simulink model "DualSixPhaseInverter"  (R2018b)
settings: Solver=ode23tb  StartTime=0.0  StopTime=0.06  MaxStep=1e-6  RelTol=1e-4
InitFcn:
  | Vm = 100;
  | f = 100;
  | Vdc1 = 200;
  | Vdc2 = 200;
  | ratio = Vdc1 / Vdc2;
  | tpwm = 1e-4;
  | Td = 2e-6;
  | R = 10;
  | L = 20e-3;
  | Vf = 1;
  | Vfd = 1;
libraries: powerlib x33, powerlib_meascontrol x24, simulink_extras x2, simulink x2
settings Model: Creator=chenhao  LastModifiedBy=chenhao

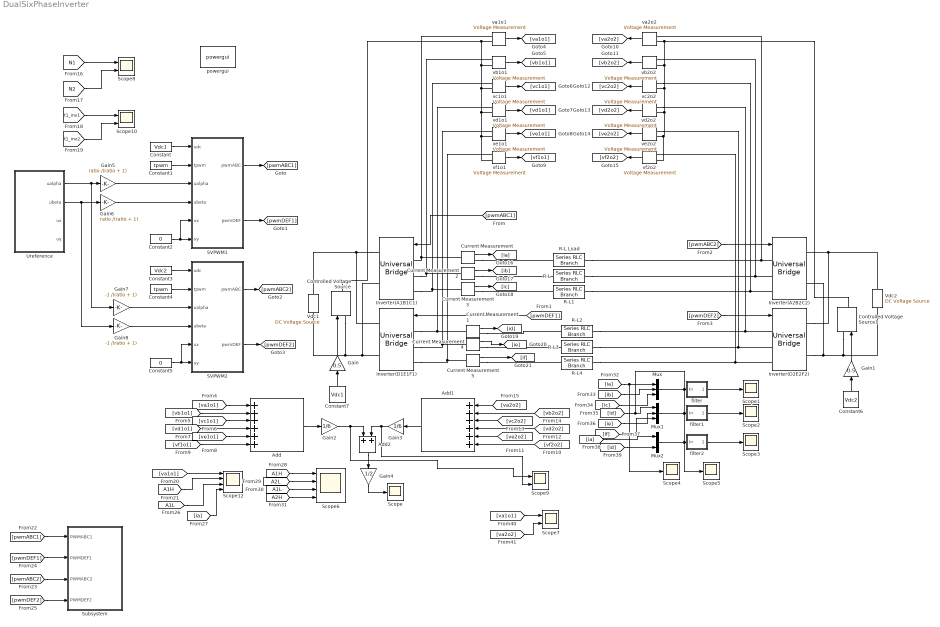
== system DualSixPhaseInverter ==
  Add : Sum  Inputs=++++++
  Add1 : Sum  Inputs=++++++
  Add2 : Sum
  Constant : Constant  Value=Vdc1
  Constant1 : Constant  Value=tpwm
  Constant2 : Constant  Value=0
  Constant3 : Constant  Value=Vdc2
  Constant4 : Constant  Value=tpwm
  Constant5 : Constant  Value=0
  Constant6 : Constant  Value=Vdc2
  Constant7 : Constant  Value=Vdc1
  Controlled Voltage Source : powerlib/Electrical Sources/Controlled Voltage Source  Initialize=on  Source_Type=AC  Amplitude=0  Phase=0  Frequency=0  Measurements=None
  Controlled Voltage Source1 : powerlib/Electrical Sources/Controlled Voltage Source  Initialize=on  Source_Type=AC  Amplitude=0  Phase=0  Frequency=0  Measurements=None
  Current Measurement{,1..5} (6 alike) : powerlib/Measurements/Current Measurement  PhasorSimulation=off  OutputType=Complex  PSBequivalent=0
  Gain : Gain  Gain=0.5
  Gain1 : Gain  Gain=0.5
  Gain2 : Gain  Gain=1/6
  Gain3 : Gain  Gain=1/6
  Gain4 : Gain  Gain=1/2
  Gain5 : Gain  Gain=ratio /(ratio + 1)
  Gain6 : Gain  Gain=ratio /(ratio + 1)
  Gain7 : Gain  Gain=-1 /(ratio + 1)
  Gain8 : Gain  Gain=-1 /(ratio + 1)
  Inverter(A1B1C1) : powerlib/Power Electronics/Universal Bridge  Arms=3  SnubberResistance=1e5  SnubberCapacitance=inf  Device=IGBT / Diodes  Ron=1e-3  Lon=0  ForwardVoltages="[  Vf  Vfd  ]"  ForwardVoltage=0  GTOparameters=[ 10e-6 , 20e-6 ]  IGBTparameters=[ 1e-6 , 2e-6 ]  Measurements=None  Measurements_2=None  converterType=Rectifier
      settings: SourceProductName=Simscape Electrical
  Inverter(A2B2C2) : powerlib/Power Electronics/Universal Bridge  Arms=3  SnubberResistance=1e5  SnubberCapacitance=inf  Device=IGBT / Diodes  Ron=1e-3  Lon=0  ForwardVoltages="[  Vf  Vfd  ]"  ForwardVoltage=0  GTOparameters=[ 10e-6 , 20e-6 ]  IGBTparameters=[ 1e-6 , 2e-6 ]  Measurements=None  Measurements_2=None  converterType=Rectifier
      settings: SourceProductName=Simscape Electrical
  Inverter(D1E1F1) : powerlib/Power Electronics/Universal Bridge  Arms=3  SnubberResistance=1e5  SnubberCapacitance=inf  Device=IGBT / Diodes  Ron=1e-3  Lon=0  ForwardVoltages="[  Vf  Vfd  ]"  ForwardVoltage=0  GTOparameters=[ 10e-6 , 20e-6 ]  IGBTparameters=[ 1e-6 , 2e-6 ]  Measurements=None  Measurements_2=None  converterType=Rectifier
      settings: SourceProductName=Simscape Electrical
  Inverter(D2E2F2) : powerlib/Power Electronics/Universal Bridge  Arms=3  SnubberResistance=1e5  SnubberCapacitance=inf  Device=IGBT / Diodes  Ron=1e-3  Lon=0  ForwardVoltages="[  Vf  Vfd  ]"  ForwardVoltage=0  GTOparameters=[ 10e-6 , 20e-6 ]  IGBTparameters=[ 1e-6 , 2e-6 ]  Measurements=None  Measurements_2=None  converterType=Rectifier
      settings: SourceProductName=Simscape Electrical
  Mux : Mux  Inputs=3
  Mux1 : Mux  Inputs=3
  Mux2 : Mux  Inputs=2
  R-L{,1..4} (5 alike) : powerlib/Elements/Series RLC Branch  LConnTagsString=__new0  RConnTagsString=__new0  BranchType=RL  Resistance=R  Inductance=L  SetiL0=off  InitialCurrent=0  Capacitance=[]  Setx0=off  InitialVoltage=0  Measurements=None
      settings: SourceProductName=Simscape Electrical
  R-L Load : powerlib/Elements/Series RLC Branch  LConnTagsString=__new0  RConnTagsString=__new0  BranchType=RL  Resistance=R  Inductance=L  SetiL0=off  InitialCurrent=0  Capacitance=[]  Setx0=off  InitialVoltage=0  Measurements=None
      settings: SourceProductName=Simscape Electrical
  SVPWM1 : Subsystem
  SVPWM2 : Subsystem
  Scope{,1..5} (6 alike) : Scope
  Scope{7..10} (4 alike) : Scope  NumInputPorts=2
  Scope12 : Scope  NumInputPorts=4
  Scope6 : Scope  NumInputPorts=4
  Subsystem : Subsystem
  Ureference : Subsystem
  Vdc1 : powerlib/Electrical Sources/DC Voltage Source  Amplitude=Vdc1  Measurements=None
      settings: SourceProductName=Simscape Electrical
  Vdc2 : powerlib/Electrical Sources/DC Voltage Source  Amplitude=Vdc2  Measurements=None
      settings: SourceProductName=Simscape Electrical
  filter : Subsystem
  filter1 : Subsystem
  filter2 : Subsystem
  powergui : powerlib/powergui  Priority=1  SimulationMode=Continuous  SampleTime=50e-6  frequency=60  Iterations=50  frequencyindice=0  Pbase=100e6  ErrMax=1e-4  UnitsV=kV  UnitsW=MW  buscounter=0  FunctionMessages=off  echomessages=off  EnableUseOfTLC=off  CurrentSourceSwitches=on  DisableSnubberDevices=off  DisableRonSwitches=off  DisableVfSwitches=off  DisplayEquations=off  SolverType=Tustin/Backward Euler (TBE)  Interpol=off  ExternalGateDelay=off  methode=off  Ts=100  x0status=blocks  SPID=off  SwTol=0  HookPort=off  RestoreLinks=warning  ResistiveCurrentMeasurement=off  Frange=[0:2:500]  Ylog=off  Xlog=on  ShowGrid=off  save=off  variable=ZData  structure=iA  ZoomFFT=off  StartTime=0.02  cycles=2  DisplayStyle=1  fundamental=100  FreqAxis=off  MaxFrequency=2000  frequencyindicesteady=1  RmsSteady=1  display=off
  va1o1 : powerlib/Measurements/Voltage Measurement  PhasorSimulation=off  OutputType=Complex  PSBequivalent=0
  va2o2 : powerlib/Measurements/Voltage Measurement  PhasorSimulation=off  OutputType=Complex  PSBequivalent=0
  vb1o1 : powerlib/Measurements/Voltage Measurement  PhasorSimulation=off  OutputType=Complex  PSBequivalent=0
  vb2o2 : powerlib/Measurements/Voltage Measurement  PhasorSimulation=off  OutputType=Complex  PSBequivalent=0
  vc1o1 : powerlib/Measurements/Voltage Measurement  PhasorSimulation=off  OutputType=Complex  PSBequivalent=0
  vc2o2 : powerlib/Measurements/Voltage Measurement  PhasorSimulation=off  OutputType=Complex  PSBequivalent=0
  vd1o1 : powerlib/Measurements/Voltage Measurement  PhasorSimulation=off  OutputType=Complex  PSBequivalent=0
  vd2o2 : powerlib/Measurements/Voltage Measurement  PhasorSimulation=off  OutputType=Complex  PSBequivalent=0
  ve1o1 : powerlib/Measurements/Voltage Measurement  PhasorSimulation=off  OutputType=Complex  PSBequivalent=0
  ve2o2 : powerlib/Measurements/Voltage Measurement  PhasorSimulation=off  OutputType=Complex  PSBequivalent=0
  vf1o1 : powerlib/Measurements/Voltage Measurement  PhasorSimulation=off  OutputType=Complex  PSBequivalent=0
  vf2o2 : powerlib/Measurements/Voltage Measurement  PhasorSimulation=off  OutputType=Complex  PSBequivalent=0
  wires:
  Constant/1 -> SVPWM1/1(udc)
  Constant1/1 -> SVPWM1/2(tpwm)
  Constant2/1 -> SVPWM1/6(uy), SVPWM1/5(ux)
  [pwmDEF1] -> Inverter(D1E1F1)/1
  [pwmABC1] -> Inverter(A1B1C1)/1
  Constant3/1 -> SVPWM2/1(udc)
  Constant4/1 -> SVPWM2/2(tpwm)
  Constant5/1 -> SVPWM2/5(ux), SVPWM2/6(uy)
  SVPWM2/1(pwmABC) -> [pwmABC2]
  Gain/1 -> Controlled Voltage Source/1
  Gain1/1 -> Controlled Voltage Source1/1
  va1o1/1 -> [va1o1]
  vb1o1/1 -> [vb1o1]
  vc1o1/1 -> [vc1o1]
  vd1o1/1 -> [vd1o1]
  ve1o1/1 -> [ve1o1]
  vf1o1/1 -> [vf1o1]
  vf2o2/1 -> [vf2o2]
  ve2o2/1 -> [ve2o2]
  vd2o2/1 -> [vd2o2]
  vc2o2/1 -> [vc2o2]
  vb2o2/1 -> [vb2o2]
  va2o2/1 -> [va2o2]
  [va1o1] -> Add/1
  [vb1o1] -> Add/2
  [vc1o1] -> Add/3
  [vd1o1] -> Add/4
  [ve1o1] -> Add/5
  [vf1o1] -> Add/6
  Add/1 -> Gain2/1
  Add1/1 -> Gain3/1
  [va2o2] -> Add1/1
  [vb2o2] -> Add1/2
  [vc2o2] -> Add1/3
  [vd2o2] -> Add1/4
  [ve2o2] -> Add1/5
  [vf2o2] -> Add1/6
  Add2/1 -> Gain4/1
  Gain4/1 -> Scope/1
  Ureference/1(ualpha) -> Gain7/1, Gain5/1
  Gain5/1 -> SVPWM1/3(ualpha)
  Ureference/2(ubeta) -> Gain8/1, Gain6/1
  Gain6/1 -> SVPWM1/4(ubeta)
  Mux/1 -> filter/1(In)
  filter/1(Out) -> Scope1/1
  Mux1/1 -> filter1/1(In)
  filter1/1(Out) -> Scope2/1
  Mux2/1 -> filter2/1(In)
  filter2/1(Out) -> Scope3/1
  [pwmABC2] -> Inverter(A2B2C2)/1
  [pwmDEF2] -> Inverter(D2E2F2)/1
  Gain8/1 -> SVPWM2/4(ubeta)
  Gain7/1 -> SVPWM2/3(ualpha)
  SVPWM1/1(pwmABC) -> [pwmABC1]
  [N1] -> Scope8/1
  [N2] -> Scope8/2
  SVPWM2/2(pwmDEF) -> [pwmDEF2]
  SVPWM1/2(pwmDEF) -> [pwmDEF1]
  Gain3/1 -> Scope9/2, Add2/2
  Gain2/1 -> Scope9/1, Add2/1
  Constant6/1 -> Gain1/1
  Constant7/1 -> Gain/1
  [t1_inv1] -> Scope10/1
  [t1_inv2] -> Scope10/2
  [va1o1] -> Scope12/1
  [A1H] -> Scope12/2
  [pwmABC1] -> Subsystem/1(PWMABC1)
  [pwmABC2] -> Subsystem/3(PWMABC2)
  [pwmDEF1] -> Subsystem/2(PWMDEF1)
  [pwmDEF2] -> Subsystem/4(PWMDEF2)
  [A1L] -> Scope12/3
  Current Measurement/1 -> [ia]
  Current Measurement2/1 -> [ib]
  Current Measurement3/1 -> [ic]
  Current Measurement1/1 -> [id]
  Current Measurement4/1 -> [ie]
  Current Measurement5/1 -> [if]
  [ia] -> Scope12/4
  [A1H] -> Scope6/1
  [A2L] -> Scope6/2
  [A1L] -> Scope6/3
  [A2H] -> Scope6/4
  [ia] -> Scope4/1, Mux/1
  [ib] -> Mux/2
  [ic] -> Mux/3
  [id] -> Scope5/1, Mux1/1
  [ie] -> Mux1/2
  [if] -> Mux1/3
  [ia] -> Mux2/1
  [id] -> Mux2/2
  [va1o1] -> Scope7/1
  [va2o2] -> Scope7/2
  connections:
  Inverter(A1B1C1)/RConn2 -- Vdc1/LConn1 -- Controlled Voltage Source/LConn1 -- Inverter(D1E1F1)/RConn2
  Inverter(D1E1F1)/LConn1 -- vd1o1/LConn1 -- Current Measurement1/LConn1
  Inverter(A1B1C1)/LConn1 -- Current Measurement/LConn1 -- va1o1/LConn1
  Inverter(A1B1C1)/RConn1 -- Vdc1/RConn1 -- Inverter(D1E1F1)/RConn1
  Inverter(D1E1F1)/LConn2 -- Current Measurement4/LConn1 -- ve1o1/LConn1
  Inverter(D1E1F1)/LConn3 -- Current Measurement5/LConn1 -- vf1o1/LConn1
  Inverter(A1B1C1)/LConn3 -- Current Measurement3/LConn1 -- vc1o1/LConn1
  Inverter(A1B1C1)/LConn2 -- Current Measurement2/LConn1 -- vb1o1/LConn1
  Inverter(D2E2F2)/RConn2 -- Vdc2/LConn1 -- Controlled Voltage Source1/LConn1 -- Inverter(A2B2C2)/RConn2
  Inverter(D2E2F2)/RConn1 -- Vdc2/RConn1 -- Inverter(A2B2C2)/RConn1
  vc2o2/LConn1 -- Inverter(A2B2C2)/LConn3 -- R-L1/RConn1
  Inverter(A2B2C2)/LConn2 -- R-L/RConn1 -- vb2o2/LConn1
  Inverter(A2B2C2)/LConn1 -- R-L Load/RConn1 -- va2o2/LConn1
  vd2o2/LConn1 -- Inverter(D2E2F2)/LConn1 -- R-L2/RConn1
  ve2o2/LConn1 -- Inverter(D2E2F2)/LConn2 -- R-L3/RConn1
  vf2o2/LConn1 -- R-L4/RConn1 -- Inverter(D2E2F2)/LConn3
  va1o1/LConn2 -- vf1o1/LConn2 -- ve1o1/LConn2 -- vd1o1/LConn2 -- vc1o1/LConn2 -- vb1o1/LConn2 -- Controlled Voltage Source/RConn1
  va2o2/LConn2 -- vf2o2/LConn2 -- ve2o2/LConn2 -- vd2o2/LConn2 -- vc2o2/LConn2 -- vb2o2/LConn2 -- Controlled Voltage Source1/RConn1
  Current Measurement/RConn1 -- R-L Load/LConn1
  Current Measurement1/RConn1 -- R-L2/LConn1
  Current Measurement2/RConn1 -- R-L/LConn1
  Current Measurement3/RConn1 -- R-L1/LConn1
  Current Measurement4/RConn1 -- R-L3/LConn1
  Current Measurement5/RConn1 -- R-L4/LConn1

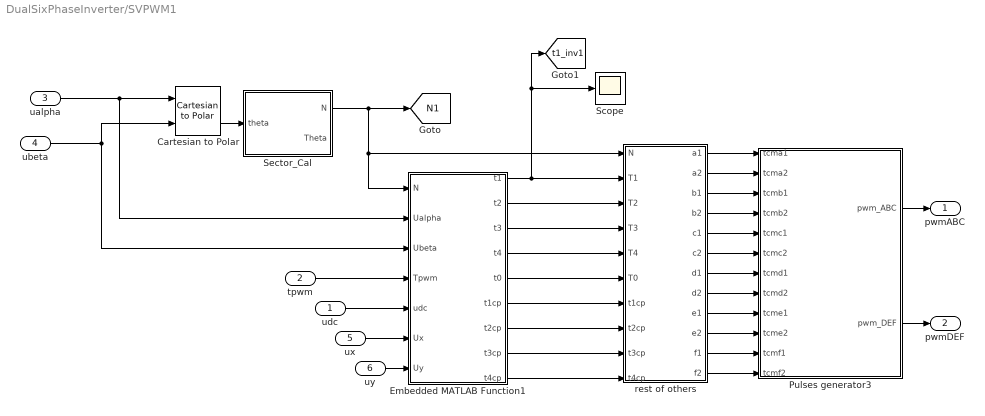
== system DualSixPhaseInverter/SVPWM1 ==
  udc : Inport
  tpwm : Inport  Port=2
  ualpha : Inport  Port=3
  ubeta : Inport  Port=4
  ux : Inport  Port=5
  uy : Inport  Port=6
  Cartesian to Polar : simulink_extras/Transformations/Cartesian to Polar
      settings: SourceProductName=Simulink
  Embedded MATLAB Function1 : MATLAB Function  TreatAsAtomicUnit=on
  Pulses generator3 : Subsystem
  Scope : Scope
  Sector_Cal : Subsystem
  rest of others : MATLAB Function  TreatAsAtomicUnit=on
  pwmABC : Outport
  pwmDEF : Outport  Port=2
  tag scope: N1=global, t1_inv1=global
  wires:
  tpwm/1 -> Embedded MATLAB Function1/4(Tpwm)
  ubeta/1 -> Cartesian to Polar/2, Embedded MATLAB Function1/3(Ubeta)
  ualpha/1 -> Cartesian to Polar/1, Embedded MATLAB Function1/2(Ualpha)
  ux/1 -> Embedded MATLAB Function1/6(Ux)
  uy/1 -> Embedded MATLAB Function1/7(Uy)
  udc/1 -> Embedded MATLAB Function1/5(udc)
  rest of others/12(f2) -> Pulses generator3/12(tcmf2)
  rest of others/11(f1) -> Pulses generator3/11(tcmf1)
  rest of others/9(e1) -> Pulses generator3/9(tcme1)
  rest of others/8(d2) -> Pulses generator3/8(tcmd2)
  rest of others/10(e2) -> Pulses generator3/10(tcme2)
  rest of others/2(a2) -> Pulses generator3/2(tcma2)
  rest of others/6(c2) -> Pulses generator3/6(tcmc2)
  rest of others/4(b2) -> Pulses generator3/4(tcmb2)
  rest of others/5(c1) -> Pulses generator3/5(tcmc1)
  rest of others/7(d1) -> Pulses generator3/7(tcmd1)
  rest of others/3(b1) -> Pulses generator3/3(tcmb1)
  rest of others/1(a1) -> Pulses generator3/1(tcma1)
  Embedded MATLAB Function1/1(t1) -> [t1_inv1], Scope/1, rest of others/2(T1)
  Embedded MATLAB Function1/2(t2) -> rest of others/3(T2)
  Embedded MATLAB Function1/3(t3) -> rest of others/4(T3)
  Embedded MATLAB Function1/4(t4) -> rest of others/5(T4)
  Embedded MATLAB Function1/5(t0) -> rest of others/6(T0)
  Embedded MATLAB Function1/6(t1cp) -> rest of others/7(t1cp)
  Embedded MATLAB Function1/7(t2cp) -> rest of others/8(t2cp)
  Embedded MATLAB Function1/8(t3cp) -> rest of others/9(t3cp)
  Embedded MATLAB Function1/9(t4cp) -> rest of others/10(t4cp)
  Cartesian to Polar/2 -> Sector_Cal/1(theta)
  Sector_Cal/1(N) -> [N1], rest of others/1(N), Embedded MATLAB Function1/1(N)
  Pulses generator3/1(pwm_ABC) -> pwmABC/1
  Pulses generator3/2(pwm_DEF) -> pwmDEF/1

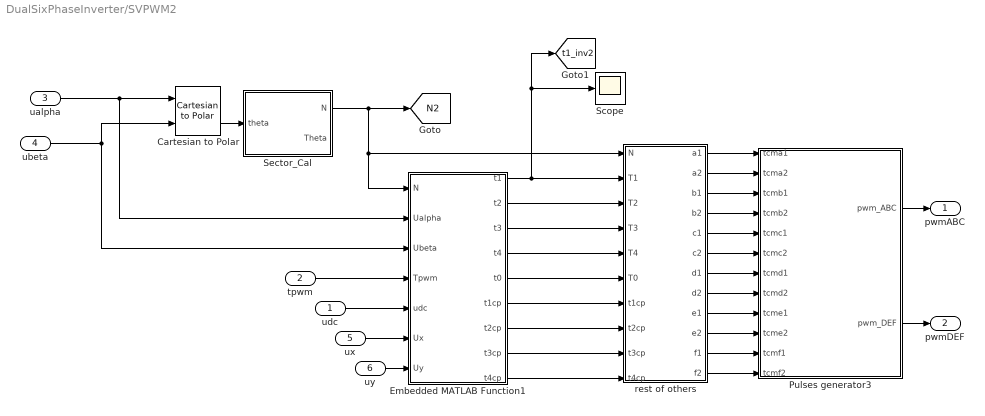
== system DualSixPhaseInverter/SVPWM2 ==
  udc : Inport
  tpwm : Inport  Port=2
  ualpha : Inport  Port=3
  ubeta : Inport  Port=4
  ux : Inport  Port=5
  uy : Inport  Port=6
  Cartesian to Polar : simulink_extras/Transformations/Cartesian to Polar
      settings: SourceProductName=Simulink
  Embedded MATLAB Function1 : MATLAB Function  TreatAsAtomicUnit=on
  Pulses generator3 : Subsystem
  Scope : Scope
  Sector_Cal : Subsystem
  rest of others : MATLAB Function  TreatAsAtomicUnit=on
  pwmABC : Outport
  pwmDEF : Outport  Port=2
  tag scope: N2=global, t1_inv2=global
  wires:
  Pulses generator3/2(pwm_DEF) -> pwmDEF/1
  Pulses generator3/1(pwm_ABC) -> pwmABC/1
  Sector_Cal/1(N) -> [N2], Embedded MATLAB Function1/1(N), rest of others/1(N)
  Cartesian to Polar/2 -> Sector_Cal/1(theta)
  Embedded MATLAB Function1/9(t4cp) -> rest of others/10(t4cp)
  Embedded MATLAB Function1/8(t3cp) -> rest of others/9(t3cp)
  Embedded MATLAB Function1/7(t2cp) -> rest of others/8(t2cp)
  Embedded MATLAB Function1/6(t1cp) -> rest of others/7(t1cp)
  Embedded MATLAB Function1/5(t0) -> rest of others/6(T0)
  Embedded MATLAB Function1/4(t4) -> rest of others/5(T4)
  Embedded MATLAB Function1/3(t3) -> rest of others/4(T3)
  Embedded MATLAB Function1/2(t2) -> rest of others/3(T2)
  Embedded MATLAB Function1/1(t1) -> rest of others/2(T1), [t1_inv2], Scope/1
  rest of others/1(a1) -> Pulses generator3/1(tcma1)
  rest of others/3(b1) -> Pulses generator3/3(tcmb1)
  rest of others/7(d1) -> Pulses generator3/7(tcmd1)
  rest of others/5(c1) -> Pulses generator3/5(tcmc1)
  rest of others/4(b2) -> Pulses generator3/4(tcmb2)
  rest of others/6(c2) -> Pulses generator3/6(tcmc2)
  rest of others/2(a2) -> Pulses generator3/2(tcma2)
  rest of others/10(e2) -> Pulses generator3/10(tcme2)
  rest of others/8(d2) -> Pulses generator3/8(tcmd2)
  rest of others/9(e1) -> Pulses generator3/9(tcme1)
  rest of others/11(f1) -> Pulses generator3/11(tcmf1)
  rest of others/12(f2) -> Pulses generator3/12(tcmf2)
  udc/1 -> Embedded MATLAB Function1/5(udc)
  uy/1 -> Embedded MATLAB Function1/7(Uy)
  ux/1 -> Embedded MATLAB Function1/6(Ux)
  ualpha/1 -> Embedded MATLAB Function1/2(Ualpha), Cartesian to Polar/1
  ubeta/1 -> Embedded MATLAB Function1/3(Ubeta), Cartesian to Polar/2
  tpwm/1 -> Embedded MATLAB Function1/4(Tpwm)

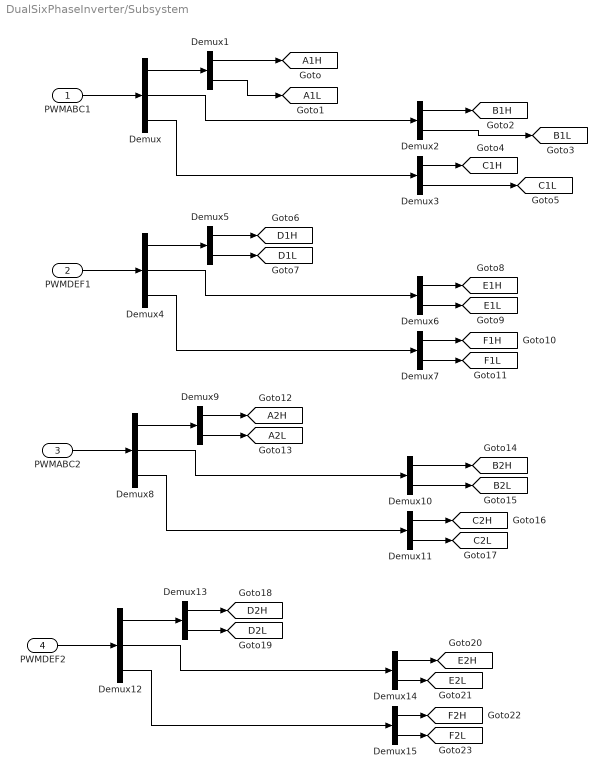
== system DualSixPhaseInverter/Subsystem ==
  PWMABC1 : Inport
  PWMDEF1 : Inport  Port=2
  PWMABC2 : Inport  Port=3
  PWMDEF2 : Inport  Port=4
  Demux{,4,8,12} (4 alike) : Demux  Outputs=3
  Demux{1..3,5..7,9..11,13..15} (12 alike) : Demux  Outputs=2
  tag scope: A1H=global, A1L=global, A2H=global, A2L=global, B1H=global, B1L=global, B2H=global, B2L=global, C1H=global, C1L=global, C2H=global, C2L=global, D1H=global, D1L=global, D2H=global, D2L=global, E1H=global, E1L=global, E2H=global, E2L=global, F1H=global, F1L=global, F2H=global, F2L=global
  wires:
  PWMABC1/1 -> Demux/1
  Demux/1 -> Demux1/1
  Demux/2 -> Demux2/1
  Demux/3 -> Demux3/1
  Demux4/3 -> Demux7/1
  Demux4/2 -> Demux6/1
  Demux4/1 -> Demux5/1
  PWMDEF1/1 -> Demux4/1
  PWMABC2/1 -> Demux8/1
  Demux8/1 -> Demux9/1
  Demux8/2 -> Demux10/1
  Demux8/3 -> Demux11/1
  Demux12/3 -> Demux15/1
  Demux12/2 -> Demux14/1
  Demux12/1 -> Demux13/1
  PWMDEF2/1 -> Demux12/1
  Demux1/1 -> [A1H]
  Demux1/2 -> [A1L]
  Demux2/1 -> [B1H]
  Demux2/2 -> [B1L]
  Demux3/1 -> [C1H]
  Demux3/2 -> [C1L]
  Demux5/1 -> [D1H]
  Demux5/2 -> [D1L]
  Demux6/1 -> [E1H]
  Demux6/2 -> [E1L]
  Demux7/1 -> [F1H]
  Demux7/2 -> [F1L]
  Demux9/1 -> [A2H]
  Demux9/2 -> [A2L]
  Demux10/1 -> [B2H]
  Demux10/2 -> [B2L]
  Demux11/1 -> [C2H]
  Demux11/2 -> [C2L]
  Demux13/1 -> [D2H]
  Demux13/2 -> [D2L]
  Demux14/1 -> [E2H]
  Demux14/2 -> [E2L]
  Demux15/1 -> [F2H]
  Demux15/2 -> [F2L]

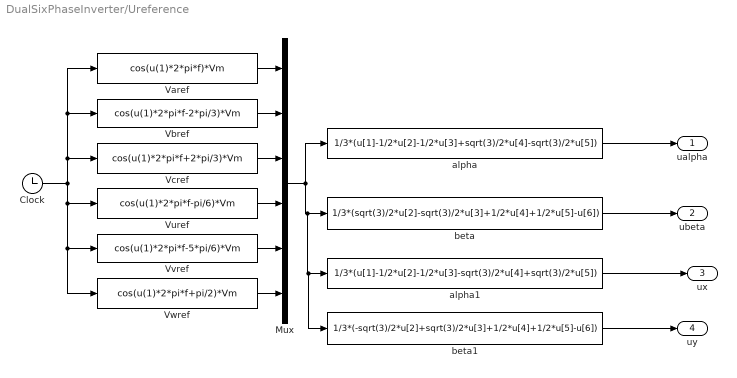
== system DualSixPhaseInverter/Ureference ==
  Clock : Clock
  Mux : Mux  Inputs=6
  Varef : Fcn  Expr=cos(u(1)*2*pi*f)*Vm
  Vbref : Fcn  Expr=cos(u(1)*2*pi*f-2*pi/3)*Vm
  Vcref : Fcn  Expr=cos(u(1)*2*pi*f+2*pi/3)*Vm
  Vuref : Fcn  Expr=cos(u(1)*2*pi*f-pi/6)*Vm
  Vvref : Fcn  Expr=cos(u(1)*2*pi*f-5*pi/6)*Vm
  Vwref : Fcn  Expr=cos(u(1)*2*pi*f+pi/2)*Vm
  alpha : Fcn  Expr=1/3*(u[1]-1/2*u[2]-1/2*u[3]+sqrt(3)/2*u[4]-sqrt(3)/2*u[5])
  alpha1 : Fcn  Expr=1/3*(u[1]-1/2*u[2]-1/2*u[3]-sqrt(3)/2*u[4]+sqrt(3)/2*u[5])
  beta : Fcn  Expr=1/3*(sqrt(3)/2*u[2]-sqrt(3)/2*u[3]+1/2*u[4]+1/2*u[5]-u[6])
  beta1 : Fcn  Expr=1/3*(-sqrt(3)/2*u[2]+sqrt(3)/2*u[3]+1/2*u[4]+1/2*u[5]-u[6])
  ualpha : Outport
  ubeta : Outport  Port=2
  ux : Outport  Port=3
  uy : Outport  Port=4
  wires:
  Vwref/1 -> Mux/6
  Vuref/1 -> Mux/4
  Vbref/1 -> Mux/2
  Vvref/1 -> Mux/5
  Varef/1 -> Mux/1
  Vcref/1 -> Mux/3
  Mux/1 -> alpha/1, beta1/1, alpha1/1, beta/1
  Clock/1 -> Varef/1, Vbref/1, Vcref/1, Vwref/1, Vvref/1, Vuref/1
  alpha/1 -> ualpha/1
  beta/1 -> ubeta/1
  alpha1/1 -> ux/1
  beta1/1 -> uy/1

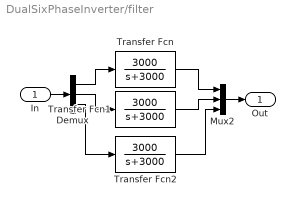
== system DualSixPhaseInverter/filter ==
  In : Inport
  Demux : Demux  Outputs=3
  Mux2 : Mux  Inputs=3
  Transfer Fcn : TransferFcn  Numerator=[3000]  Denominator=[1 3000]
  Transfer Fcn1 : TransferFcn  Numerator=[3000]  Denominator=[1 3000]
  Transfer Fcn2 : TransferFcn  Numerator=[3000]  Denominator=[1 3000]
  Out : Outport
  wires:
  Demux/1 -> Transfer Fcn/1
  Demux/2 -> Transfer Fcn1/1
  Transfer Fcn1/1 -> Mux2/2
  Transfer Fcn/1 -> Mux2/1
  In/1 -> Demux/1
  Mux2/1 -> Out/1
  Demux/3 -> Transfer Fcn2/1
  Transfer Fcn2/1 -> Mux2/3

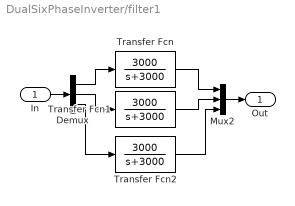
== system DualSixPhaseInverter/filter1 ==
  In : Inport
  Demux : Demux  Outputs=3
  Mux2 : Mux  Inputs=3
  Transfer Fcn : TransferFcn  Numerator=[3000]  Denominator=[1 3000]
  Transfer Fcn1 : TransferFcn  Numerator=[3000]  Denominator=[1 3000]
  Transfer Fcn2 : TransferFcn  Numerator=[3000]  Denominator=[1 3000]
  Out : Outport
  wires:
  Transfer Fcn2/1 -> Mux2/3
  Demux/3 -> Transfer Fcn2/1
  Mux2/1 -> Out/1
  In/1 -> Demux/1
  Transfer Fcn/1 -> Mux2/1
  Transfer Fcn1/1 -> Mux2/2
  Demux/2 -> Transfer Fcn1/1
  Demux/1 -> Transfer Fcn/1

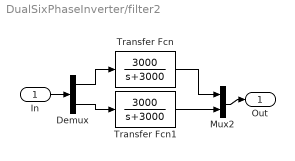
== system DualSixPhaseInverter/filter2 ==
  In : Inport
  Demux : Demux  Outputs=2
  Mux2 : Mux  Inputs=2
  Transfer Fcn : TransferFcn  Numerator=[3000]  Denominator=[1 3000]
  Transfer Fcn1 : TransferFcn  Numerator=[3000]  Denominator=[1 3000]
  Out : Outport
  wires:
  Demux/1 -> Transfer Fcn/1
  Demux/2 -> Transfer Fcn1/1
  Transfer Fcn1/1 -> Mux2/2
  Transfer Fcn/1 -> Mux2/1
  In/1 -> Demux/1
  Mux2/1 -> Out/1

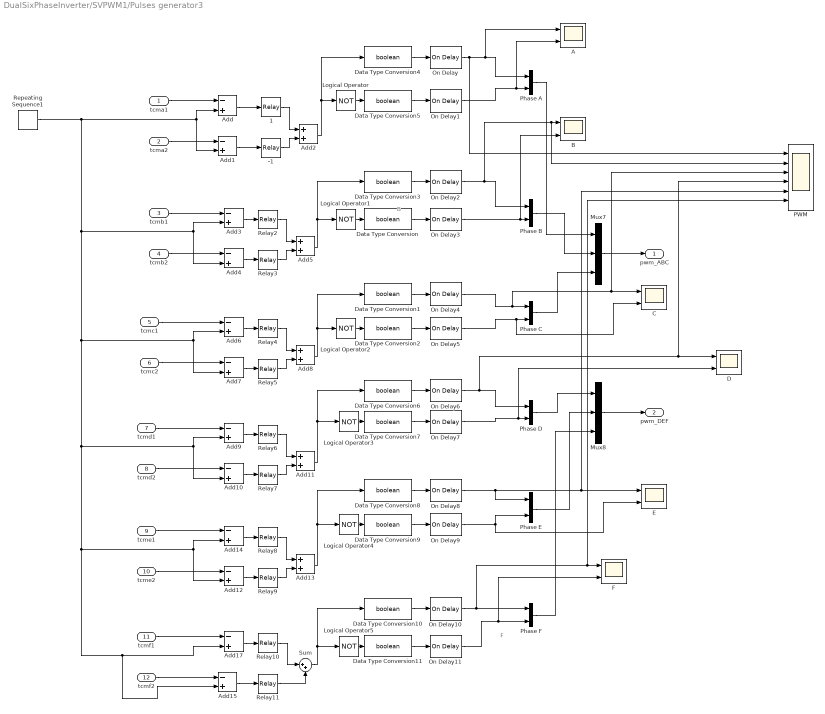
== system DualSixPhaseInverter/SVPWM1/Pulses generator3 ==
  note: B
  note: F
  tcma1 : Inport
  tcma2 : Inport  Port=2
  tcmb1 : Inport  Port=3
  tcmb2 : Inport  Port=4
  tcmc1 : Inport  Port=5
  tcmc2 : Inport  Port=6
  tcmd1 : Inport  Port=7
  tcmd2 : Inport  Port=8
  tcme1 : Inport  Port=9
  tcme2 : Inport  Port=10
  tcmf1 : Inport  Port=11
  tcmf2 : Inport  Port=12
  -1 : Relay  OnOutputValue=-1
  1 : Relay
  A : Scope  NumInputPorts=2
  Add{,1,3..4,6..7,9..10,12,14..15,17} (12 alike) : Sum  Inputs=-+
  Add{2,5,8,11,13} (5 alike) : Sum
  B : Scope  NumInputPorts=2
  C : Scope  NumInputPorts=2
  D : Scope  NumInputPorts=2
  Data Type Conversion{,1..11} (12 alike) : DataTypeConversion  OutDataTypeStr=boolean
  E : Scope  NumInputPorts=2
  F : Scope  NumInputPorts=2
  Logical Operator{,1..5} (6 alike) : Logic  Operator=NOT  AllPortsSameDT=off  OutDataTypeStr=boolean
  Mux7 : Mux  Inputs=3
  Mux8 : Mux  Inputs=3
  On Delay{,1..11} (12 alike) : powerlib_meascontrol/Logic/On Delay  DelayType=On delay  delay=Td  ic=0  Ts=0
      settings: SourceProductName=Simscape Power Systems
  PWM : Scope  NumInputPorts=6
  Phase A : Mux  Inputs=2
  Phase B : Mux  Inputs=2
  Phase C : Mux  Inputs=2
  Phase D : Mux  Inputs=2
  Phase E : Mux  Inputs=2
  Phase F : Mux  Inputs=2
  Relay{2,4,6,8,10} (5 alike) : Relay
  Relay{3,5,7,9,11} (5 alike) : Relay  OnOutputValue=-1
  Repeating Sequence1 : simulink/Sources/Repeating Sequence  rep_seq_t=[0 tpwm]  rep_seq_y=[0 tpwm]
  Sum : Sum  Inputs=|++
  pwm_ABC : Outport
  pwm_DEF : Outport  Port=2
  wires:
  On Delay11/1 -> F/2, Phase F/2
  Data Type Conversion11/1 -> On Delay11/1
  On Delay10/1 -> PWM/6, F/1, Phase F/1
  Data Type Conversion10/1 -> On Delay10/1
  On Delay9/1 -> E/2, Phase E/2
  Data Type Conversion9/1 -> On Delay9/1
  On Delay8/1 -> Phase E/1, PWM/5, E/1
  Data Type Conversion8/1 -> On Delay8/1
  On Delay7/1 -> D/2, Phase D/2
  Data Type Conversion7/1 -> On Delay7/1
  On Delay6/1 -> PWM/4, D/1, Phase D/1
  Data Type Conversion6/1 -> On Delay6/1
  On Delay5/1 -> C/2, Phase C/2
  Data Type Conversion2/1 -> On Delay5/1
  On Delay4/1 -> PWM/3, C/1, Phase C/1
  Data Type Conversion1/1 -> On Delay4/1
  On Delay2/1 -> PWM/2, B/1, Phase B/1
  On Delay3/1 -> B/2, Phase B/2
  Data Type Conversion/1 -> On Delay3/1
  Data Type Conversion3/1 -> On Delay2/1
  On Delay1/1 -> A/2, Phase A/2
  Data Type Conversion5/1 -> On Delay1/1
  On Delay/1 -> A/1, Phase A/1, PWM/1
  Data Type Conversion4/1 -> On Delay/1
  Logical Operator3/1 -> Data Type Conversion7/1
  Logical Operator2/1 -> Data Type Conversion2/1
  Logical Operator/1 -> Data Type Conversion5/1
  Logical Operator1/1 -> Data Type Conversion/1
  Logical Operator4/1 -> Data Type Conversion9/1
  Add5/1 -> Logical Operator1/1, Data Type Conversion3/1
  Add2/1 -> Logical Operator/1, Data Type Conversion4/1
  Mux8/1 -> pwm_DEF/1
  Mux7/1 -> pwm_ABC/1
  Sum/1 -> Data Type Conversion10/1, Logical Operator5/1
  Add13/1 -> Data Type Conversion8/1, Logical Operator4/1
  Add11/1 -> Data Type Conversion6/1, Logical Operator3/1
  Add8/1 -> Data Type Conversion1/1, Logical Operator2/1
  Logical Operator5/1 -> Data Type Conversion11/1
  tcmf2/1 -> Add15/1
  Relay11/1 -> Sum/2
  Relay10/1 -> Sum/1
  Add17/1 -> Relay10/1
  tcmf1/1 -> Add17/1
  tcme2/1 -> Add12/1
  Relay9/1 -> Add13/2
  Relay8/1 -> Add13/1
  Add12/1 -> Relay9/1
  Add14/1 -> Relay8/1
  tcme1/1 -> Add14/1
  tcmd2/1 -> Add10/1
  Relay7/1 -> Add11/2
  Relay6/1 -> Add11/1
  Add10/1 -> Relay7/1
  Add9/1 -> Relay6/1
  tcmd1/1 -> Add9/1
  tcmc2/1 -> Add7/1
  Relay5/1 -> Add8/2
  Relay4/1 -> Add8/1
  Add7/1 -> Relay5/1
  Add6/1 -> Relay4/1
  tcmb2/1 -> Add4/1
  Relay3/1 -> Add5/2
  Relay2/1 -> Add5/1
  Add4/1 -> Relay3/1
  Add3/1 -> Relay2/1
  tcma1/1 -> Add/1
  -1/1 -> Add2/2
  1/1 -> Add2/1
  Add1/1 -> -1/1
  Add/1 -> 1/1
  Repeating Sequence1/1 -> Add15/2, Add17/2, Add12/2, Add14/2, Add9/2, Add10/2, Add7/2, Add6/2, Add3/2, Add4/2, Add1/2, Add/2
  tcma2/1 -> Add1/1
  tcmb1/1 -> Add3/1
  tcmc1/1 -> Add6/1
  Add15/1 -> Relay11/1
  Phase A/1 -> Mux7/1
  Phase B/1 -> Mux7/2
  Phase C/1 -> Mux7/3
  Phase D/1 -> Mux8/1
  Phase E/1 -> Mux8/2
  Phase F/1 -> Mux8/3

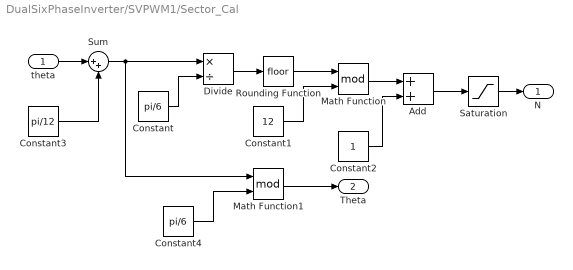
== system DualSixPhaseInverter/SVPWM1/Sector_Cal ==
  theta : Inport
  Add : Sum
  Constant : Constant  Value=pi/6
  Constant1 : Constant  Value=12
  Constant2 : Constant
  Constant3 : Constant  Value=pi/12
  Constant4 : Constant  Value=pi/6
  Divide : Product  Inputs=*/
  Math Function : Math  Operator=mod  SaturateOnIntegerOverflow=on
  Math Function1 : Math  Operator=mod  SaturateOnIntegerOverflow=on
  Rounding Function : Rounding
  Saturation : Saturate  UpperLimit=12  LowerLimit=1
  Sum : Sum  Inputs=|++
  N : Outport
  Theta : Outport  Port=2
  wires:
  Constant/1 -> Divide/2
  Divide/1 -> Rounding Function/1
  Rounding Function/1 -> Math Function/1
  Constant1/1 -> Math Function/2
  Math Function/1 -> Add/1
  Constant2/1 -> Add/2
  Add/1 -> Saturation/1
  Saturation/1 -> N/1
  theta/1 -> Sum/1
  Sum/1 -> Math Function1/1, Divide/1
  Constant3/1 -> Sum/2
  Constant4/1 -> Math Function1/2
  Math Function1/1 -> Theta/1

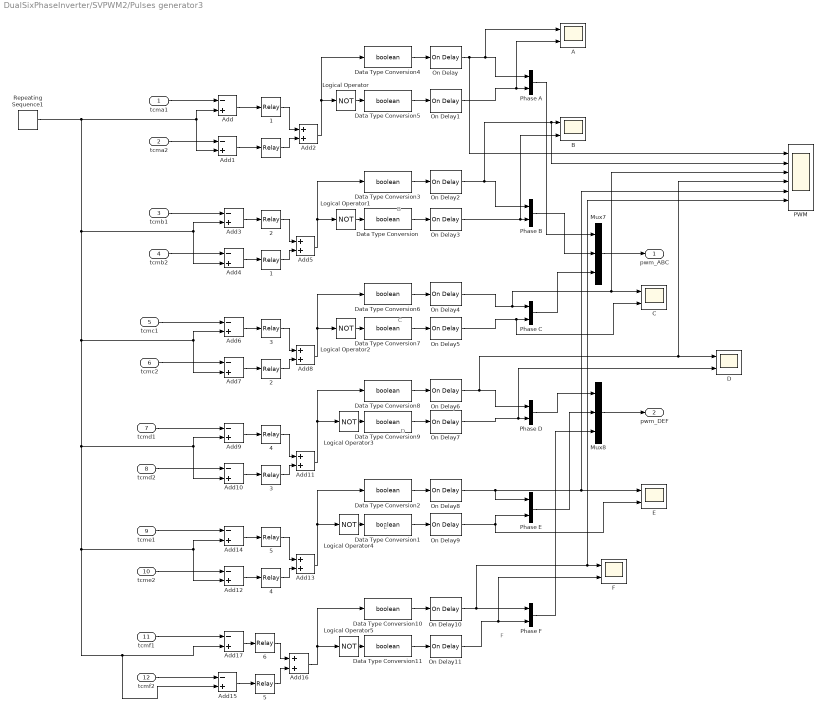
== system DualSixPhaseInverter/SVPWM2/Pulses generator3 ==
  note: F
  note: E
  note: D
  note: C
  note: B
  tcma1 : Inport
  tcma2 : Inport  Port=2
  tcmb1 : Inport  Port=3
  tcmb2 : Inport  Port=4
  tcmc1 : Inport  Port=5
  tcmc2 : Inport  Port=6
  tcmd1 : Inport  Port=7
  tcmd2 : Inport  Port=8
  tcme1 : Inport  Port=9
  tcme2 : Inport  Port=10
  tcmf1 : Inport  Port=11
  tcmf2 : Inport  Port=12
   {,1..5} (6 alike) : Relay
  {1..6} (6 alike) : Relay  OnOutputValue=0  OffOutputValue=1
  A : Scope  NumInputPorts=2
  Add{,1,3..4,6..7,9..10,12,14..15,17} (12 alike) : Sum  Inputs=-+
  Add{2,5,8,11,13,16} (6 alike) : Sum
  B : Scope  NumInputPorts=2
  C : Scope  NumInputPorts=2
  D : Scope  NumInputPorts=2
  Data Type Conversion{,1..11} (12 alike) : DataTypeConversion  OutDataTypeStr=boolean
  E : Scope  NumInputPorts=2
  F : Scope  NumInputPorts=2
  Logical Operator{,1..5} (6 alike) : Logic  Operator=NOT  AllPortsSameDT=off  OutDataTypeStr=boolean
  Mux7 : Mux  Inputs=3
  Mux8 : Mux  Inputs=3
  On Delay{,1..11} (12 alike) : powerlib_meascontrol/Logic/On Delay  DelayType=On delay  delay=Td  ic=0  Ts=0
      settings: SourceProductName=Simscape Power Systems
  PWM : Scope  NumInputPorts=6
  Phase A : Mux  Inputs=2
  Phase B : Mux  Inputs=2
  Phase C : Mux  Inputs=2
  Phase D : Mux  Inputs=2
  Phase E : Mux  Inputs=2
  Phase F : Mux  Inputs=2
  Repeating Sequence1 : simulink/Sources/Repeating Sequence  rep_seq_t=[0 tpwm]  rep_seq_y=[0 tpwm]
  pwm_ABC : Outport
  pwm_DEF : Outport  Port=2
  wires:
  Phase F/1 -> Mux8/3
  Phase E/1 -> Mux8/2
  Phase D/1 -> Mux8/1
  Phase C/1 -> Mux7/3
  Phase B/1 -> Mux7/2
  Phase A/1 -> Mux7/1
  tcmc1/1 -> Add6/1
  tcmb1/1 -> Add3/1
  tcma2/1 -> Add1/1
  Repeating Sequence1/1 -> Add/2, Add1/2, Add4/2, Add3/2, Add6/2, Add7/2, Add10/2, Add9/2, Add14/2, Add12/2, Add17/2, Add15/2
  Add/1 -> 1/1
  Add1/1 -> " "/1
  1/1 -> Add2/1
  " "/1 -> Add2/2
  tcma1/1 -> Add/1
  tcmb2/1 -> Add4/1
  tcmc2/1 -> Add7/1
  tcmd1/1 -> Add9/1
  tcmd2/1 -> Add10/1
  tcme1/1 -> Add14/1
  tcme2/1 -> Add12/1
  tcmf1/1 -> Add17/1
  tcmf2/1 -> Add15/1
  Logical Operator5/1 -> Data Type Conversion11/1
  Add8/1 -> Data Type Conversion6/1, Logical Operator2/1
  Add11/1 -> Data Type Conversion8/1, Logical Operator3/1
  Add13/1 -> Data Type Conversion2/1, Logical Operator4/1
  Add16/1 -> Data Type Conversion10/1, Logical Operator5/1
  Mux7/1 -> pwm_ABC/1
  Mux8/1 -> pwm_DEF/1
  Add2/1 -> Data Type Conversion4/1, Logical Operator/1
  Add5/1 -> Data Type Conversion3/1, Logical Operator1/1
  Logical Operator4/1 -> Data Type Conversion1/1
  Logical Operator1/1 -> Data Type Conversion/1
  Logical Operator/1 -> Data Type Conversion5/1
  Logical Operator2/1 -> Data Type Conversion7/1
  Logical Operator3/1 -> Data Type Conversion9/1
  Data Type Conversion4/1 -> On Delay/1
  On Delay/1 -> PWM/1, Phase A/1, A/1
  Data Type Conversion5/1 -> On Delay1/1
  On Delay1/1 -> Phase A/2, A/2
  Data Type Conversion3/1 -> On Delay2/1
  Data Type Conversion/1 -> On Delay3/1
  On Delay3/1 -> Phase B/2, B/2
  On Delay2/1 -> Phase B/1, B/1, PWM/2
  Data Type Conversion6/1 -> On Delay4/1
  On Delay4/1 -> Phase C/1, C/1, PWM/3
  Data Type Conversion7/1 -> On Delay5/1
  On Delay5/1 -> Phase C/2, C/2
  Data Type Conversion8/1 -> On Delay6/1
  On Delay6/1 -> Phase D/1, D/1, PWM/4
  Data Type Conversion9/1 -> On Delay7/1
  On Delay7/1 -> Phase D/2, D/2
  Data Type Conversion2/1 -> On Delay8/1
  On Delay8/1 -> E/1, PWM/5, Phase E/1
  Data Type Conversion1/1 -> On Delay9/1
  On Delay9/1 -> Phase E/2, E/2
  Data Type Conversion10/1 -> On Delay10/1
  On Delay10/1 -> Phase F/1, F/1, PWM/6
  Data Type Conversion11/1 -> On Delay11/1
  On Delay11/1 -> Phase F/2, F/2
  " 1"/1 -> Add5/2
  2/1 -> Add5/1
  Add4/1 -> " 1"/1
  Add3/1 -> 2/1
  " 2"/1 -> Add8/2
  3/1 -> Add8/1
  Add7/1 -> " 2"/1
  Add6/1 -> 3/1
  4/1 -> Add11/1
  " 3"/1 -> Add11/2
  Add10/1 -> " 3"/1
  Add9/1 -> 4/1
  Add14/1 -> 5/1
  Add12/1 -> " 4"/1
  " 4"/1 -> Add13/2
  5/1 -> Add13/1
  6/1 -> Add16/1
  " 5"/1 -> Add16/2
  Add15/1 -> " 5"/1
  Add17/1 -> 6/1

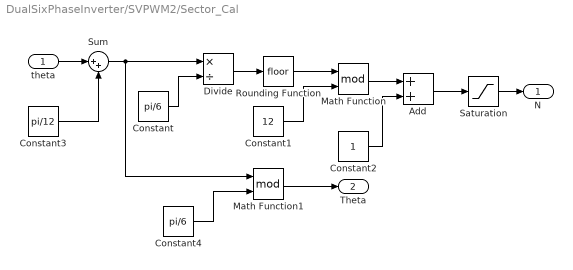
== system DualSixPhaseInverter/SVPWM2/Sector_Cal ==
  theta : Inport
  Add : Sum
  Constant : Constant  Value=pi/6
  Constant1 : Constant  Value=12
  Constant2 : Constant
  Constant3 : Constant  Value=pi/12
  Constant4 : Constant  Value=pi/6
  Divide : Product  Inputs=*/
  Math Function : Math  Operator=mod  SaturateOnIntegerOverflow=on
  Math Function1 : Math  Operator=mod  SaturateOnIntegerOverflow=on
  Rounding Function : Rounding
  Saturation : Saturate  UpperLimit=12  LowerLimit=1
  Sum : Sum  Inputs=|++
  N : Outport
  Theta : Outport  Port=2
  wires:
  Math Function1/1 -> Theta/1
  Constant4/1 -> Math Function1/2
  Constant3/1 -> Sum/2
  Sum/1 -> Divide/1, Math Function1/1
  theta/1 -> Sum/1
  Saturation/1 -> N/1
  Add/1 -> Saturation/1
  Constant2/1 -> Add/2
  Math Function/1 -> Add/1
  Constant1/1 -> Math Function/2
  Rounding Function/1 -> Math Function/1
  Divide/1 -> Rounding Function/1
  Constant/1 -> Divide/2

== matlab function DualSixPhaseInverter/SVPWM1/Embedded MATLAB Function1 ==
  data: N input; t1 output; Ualpha input; Ubeta input; Tpwm input; t2 output; t3 output; t4 output; t0 output; udc input; Ux input; Uy input; t1cp output; t2cp output; t3cp output; t4cp output
function [t1, t2, t3, t4, t0, t1cp, t2cp, t3cp, t4cp] = fcn(N, Ualpha, Ubeta, Tpwm, udc, Ux,Uy)

m=sqrt(3)/2+1/2*1i;

%等幅clarke反变换
ab44=1/3*udc*[1,m^4,m^8,m,m^5,m^9]*[1;0;0;1;0;0];
xy44=1/3*udc*[1,m^8,m^4,m^5,m,m^9]*[1;0;0;1;0;0];

ab64=1/3*udc*[1,m^4,m^8,m,m^5,m^9]*[1;1;0;1;0;0];
xy64=1/3*udc*[1,m^8,m^4,m^5,m,m^9]*[1;1;0;1;0;0];
        
ab66=1/3*udc*[1,m^4,m^8,m,m^5,m^9]*[1;1;0;1;1;0];
xy66=1/3*udc*[1,m^8,m^4,m^5,m,m^9]*[1;1;0;1;1;0];

ab26=1/3*udc*[1,m^4,m^8,m,m^5,m^9]*[0;1;0;1;1;0];
xy26=1/3*udc*[1,m^8,m^4,m^5,m,m^9]*[0;1;0;1;1;0];

ab22=1/3*udc*[1,m^4,m^8,m,m^5,m^9]*[0;1;0;0;1;0];
xy22=1/3*udc*[1,m^8,m^4,m^5,m,m^9]*[0;1;0;0;1;0];

ab32=1/3*udc*[1,m^4,m^8,m,m^5,m^9]*[0;1;1;0;1;0];
xy32=1/3*udc*[1,m^8,m^4,m^5,m,m^9]*[0;1;1;0;1;0];

ab33=1/3*udc*[1,m^4,m^8,m,m^5,m^9]*[0;1;1;0;1;1];
xy33=1/3*udc*[1,m^8,m^4,m^5,m,m^9]*[0;1;1;0;1;1];

ab13=1/3*udc*[1,m^4,m^8,m,m^5,m^9]*[0;0;1;0;1;1];
xy13=1/3*udc*[1,m^8,m^4,m^5,m,m^9]*[0;0;1;0;1;1];

ab11=1/3*udc*[1,m^4,m^8,m,m^5,m^9]*[0;0;1;0;0;1];
xy11=1/3*udc*[1,m^8,m^4,m^5,m,m^9]*[0;0;1;0;0;1];

ab51=1/3*udc*[1,m^4,m^8,m,m^5,m^9]*[1;0;1;0;0;1];
xy51=1/3*udc*[1,m^8,m^4,m^5,m,m^9]*[1;0;1;0;0;1];

ab55=1/3*udc*[1,m^4,m^8,m,m^5,m^9]*[1;0;1;1;0;1];
xy55=1/3*udc*[1,m^8,m^4,m^5,m,m^9]*[1;0;1;1;0;1];

ab45=1/3*udc*[1,m^4,m^8,m,m^5,m^9]*[1;0;0;1;0;1];
xy45=1/3*udc*[1,m^8,m^4,m^5,m,m^9]*[1;0;0;1;0;1];

switch N
    case 1
        X=[real(ab55),real(ab45),real(ab44),real(ab64);
           imag(ab55),imag(ab45),imag(ab44),imag(ab64);
           real(xy55),real(xy45),real(xy44),real(xy64);
           imag(xy55),imag(xy45),imag(xy44),imag(xy64)];

    case 2
        X=[real(ab45),real(ab44),real(ab64),real(ab66);
           imag(ab45),imag(ab44),imag(ab64),imag(ab66);
           real(xy45),real(xy44),real(xy64),real(xy66);
           imag(xy45),imag(xy44),imag(xy64),imag(xy66)];

    case 3
        X=[real(ab44),real(ab64),real(ab66),real(ab26);
           imag(ab44),imag(ab64),imag(ab66),imag(ab26);
           real(xy44),real(xy64),real(xy66),real(xy26);
           imag(xy44),imag(xy64),imag(xy66),imag(xy26)];

    case 4
        X=[real(ab64),real(ab66),real(ab26),real(ab22);
           imag(ab64),imag(ab66),imag(ab26),imag(ab22);
           real(xy64),real(xy66),real(xy26),real(xy22);
           imag(xy64),imag(xy66),imag(xy26),imag(xy22)];

    case 5
        X=[real(ab66),real(ab26),real(ab22),real(ab32);
           imag(ab66),imag(ab26),imag(ab22),imag(ab32);
           real(xy66),real(xy26),real(xy22),real(xy32);
           imag(xy66),imag(xy26),imag(xy22),imag(xy32)];

    case 6
        X=[real(ab26),real(ab22),real(ab32),real(ab33);
           imag(ab26),imag(ab22),imag(ab32),imag(ab33);
           real(xy26),real(xy22),real(xy32),real(xy33);
           imag(xy26),imag(xy22),imag(xy32),imag(xy33)];

    case 7
        X=[real(ab22),real(ab32),real(ab33),real(ab13);
           imag(ab22),imag(ab32),imag(ab33),imag(ab13);
           real(xy22),real(xy32),real(xy33),real(xy13);
           imag(xy22),imag(xy32),imag(xy33),imag(xy13)];

    case 8
        X=[real(ab32),real(ab33),real(ab13),real(ab11);
           imag(ab32),imag(ab33),imag(ab13),imag(ab11);
           real(xy32),real(xy33),real(xy13),real(xy11);
           imag(xy32),imag(xy33),imag(xy13),imag(xy11)];

    case 9
        X=[real(ab33),real(ab13),real(ab11),real(ab51);
           imag(ab33),imag(ab13),imag(ab11),imag(ab51);
           real(xy33),real(xy13),real(xy11),real(xy51);
           imag(xy33),imag(xy13),imag(xy11),imag(xy51)];

    case 10
        X=[real(ab13),real(ab11),real(ab51),real(ab55);
           imag(ab13),imag(ab11),imag(ab51),imag(ab55);
           real(xy13),real(xy11),real(xy51),real(xy55);
           imag(xy13),imag(xy11),imag(xy51),imag(xy55)];

    case 11
        X=[real(ab11),real(ab51),real(ab55),real(ab45);
           imag(ab11),imag(ab51),imag(ab55),imag(ab45);
           real(xy11),real(xy51),real(xy55),real(xy45);
           imag(xy11),imag(xy51),imag(xy55),imag(xy45)];

    case 12
        X=[real(ab51),real(ab55),real(ab45),real(ab44);
           imag(ab51),imag(ab55),imag(ab45),imag(ab44);
           real(xy51),real(xy55),real(xy45),real(xy44);
           imag(xy51),imag(xy55),imag(xy45),imag(xy44)];

    otherwise
        X=[0,0,0,0;
           0,0,0,0;
           0,0,0,0;
           0,0,0,0];

end
Y=[Ualpha;Ubeta;Ux;Uy]*Tpwm;
T = X \ Y;

% t1=T(1);
% if t1<15e-6
%     t1=15e-6;
% end
% t2=T(2);
% if t2<15e-6
%     t2=15e-6;
% end
% t3=T(3);
% if t3<1e-6
%     t3=1e-6;
% end
% t4=T(4);
% if t4<1e-6
%     t4=1e-6;
% end

t1=T(1);
t2=T(2);
t3=T(3);
t4=T(4);
t1cp = 0;
t2cp = 0;
t3cp = 0;
t4cp = 0;
% if T(1) >= 0
%     t1 = T(1);
% else
%     t1 = 0;
%     t1cp = -T(1);
% end
% if T(2) >= 0
%     t2 = T(2);
% else
%     t2 = 0;
%     t2cp = -T(2);
% end
% if T(3) >= 0
%     t3 = T(3);
% else
%     t3 = 0;
%     t3cp = -T(3);
% end
% if T(4) >= 0
%     t4 = T(4);
% else
%     t4 = 0;
%     t4cp = -T(4);
% end

Tsum=t1+t2+t3+t4;
if Tsum>Tpwm
    t1=t1*Tpwm/Tsum;
    t2=t2*Tpwm/Tsum;
    t3=t3*Tpwm/Tsum;
    t4=t4*Tpwm/Tsum;
end
t0=Tpwm-t1-t2-t3-t4;
end

== matlab function DualSixPhaseInverter/SVPWM2/Embedded MATLAB Function1 ==
  data: N input; t1 output; Ualpha input; Ubeta input; Tpwm input; t2 output; t3 output; t4 output; t0 output; udc input; Ux input; Uy input; t1cp output; t2cp output; t3cp output; t4cp output
function [t1, t2, t3, t4, t0, t1cp, t2cp, t3cp, t4cp] = fcn(N, Ualpha, Ubeta, Tpwm, udc, Ux,Uy)

m=sqrt(3)/2+1/2*1i;

%等幅clarke反变换
ab44=1/3*udc*[1,m^4,m^8,m,m^5,m^9]*[1;0;0;1;0;0];
xy44=1/3*udc*[1,m^8,m^4,m^5,m,m^9]*[1;0;0;1;0;0];

ab64=1/3*udc*[1,m^4,m^8,m,m^5,m^9]*[1;1;0;1;0;0];
xy64=1/3*udc*[1,m^8,m^4,m^5,m,m^9]*[1;1;0;1;0;0];
        
ab66=1/3*udc*[1,m^4,m^8,m,m^5,m^9]*[1;1;0;1;1;0];
xy66=1/3*udc*[1,m^8,m^4,m^5,m,m^9]*[1;1;0;1;1;0];

ab26=1/3*udc*[1,m^4,m^8,m,m^5,m^9]*[0;1;0;1;1;0];
xy26=1/3*udc*[1,m^8,m^4,m^5,m,m^9]*[0;1;0;1;1;0];

ab22=1/3*udc*[1,m^4,m^8,m,m^5,m^9]*[0;1;0;0;1;0];
xy22=1/3*udc*[1,m^8,m^4,m^5,m,m^9]*[0;1;0;0;1;0];

ab32=1/3*udc*[1,m^4,m^8,m,m^5,m^9]*[0;1;1;0;1;0];
xy32=1/3*udc*[1,m^8,m^4,m^5,m,m^9]*[0;1;1;0;1;0];

ab33=1/3*udc*[1,m^4,m^8,m,m^5,m^9]*[0;1;1;0;1;1];
xy33=1/3*udc*[1,m^8,m^4,m^5,m,m^9]*[0;1;1;0;1;1];

ab13=1/3*udc*[1,m^4,m^8,m,m^5,m^9]*[0;0;1;0;1;1];
xy13=1/3*udc*[1,m^8,m^4,m^5,m,m^9]*[0;0;1;0;1;1];

ab11=1/3*udc*[1,m^4,m^8,m,m^5,m^9]*[0;0;1;0;0;1];
xy11=1/3*udc*[1,m^8,m^4,m^5,m,m^9]*[0;0;1;0;0;1];

ab51=1/3*udc*[1,m^4,m^8,m,m^5,m^9]*[1;0;1;0;0;1];
xy51=1/3*udc*[1,m^8,m^4,m^5,m,m^9]*[1;0;1;0;0;1];

ab55=1/3*udc*[1,m^4,m^8,m,m^5,m^9]*[1;0;1;1;0;1];
xy55=1/3*udc*[1,m^8,m^4,m^5,m,m^9]*[1;0;1;1;0;1];

ab45=1/3*udc*[1,m^4,m^8,m,m^5,m^9]*[1;0;0;1;0;1];
xy45=1/3*udc*[1,m^8,m^4,m^5,m,m^9]*[1;0;0;1;0;1];

switch N
    case 1
        X=[real(ab55),real(ab45),real(ab44),real(ab64);
           imag(ab55),imag(ab45),imag(ab44),imag(ab64);
           real(xy55),real(xy45),real(xy44),real(xy64);
           imag(xy55),imag(xy45),imag(xy44),imag(xy64)];

    case 2
        X=[real(ab45),real(ab44),real(ab64),real(ab66);
           imag(ab45),imag(ab44),imag(ab64),imag(ab66);
           real(xy45),real(xy44),real(xy64),real(xy66);
           imag(xy45),imag(xy44),imag(xy64),imag(xy66)];

    case 3
        X=[real(ab44),real(ab64),real(ab66),real(ab26);
           imag(ab44),imag(ab64),imag(ab66),imag(ab26);
           real(xy44),real(xy64),real(xy66),real(xy26);
           imag(xy44),imag(xy64),imag(xy66),imag(xy26)];

    case 4
        X=[real(ab64),real(ab66),real(ab26),real(ab22);
           imag(ab64),imag(ab66),imag(ab26),imag(ab22);
           real(xy64),real(xy66),real(xy26),real(xy22);
           imag(xy64),imag(xy66),imag(xy26),imag(xy22)];

    case 5
        X=[real(ab66),real(ab26),real(ab22),real(ab32);
           imag(ab66),imag(ab26),imag(ab22),imag(ab32);
           real(xy66),real(xy26),real(xy22),real(xy32);
           imag(xy66),imag(xy26),imag(xy22),imag(xy32)];

    case 6
        X=[real(ab26),real(ab22),real(ab32),real(ab33);
           imag(ab26),imag(ab22),imag(ab32),imag(ab33);
           real(xy26),real(xy22),real(xy32),real(xy33);
           imag(xy26),imag(xy22),imag(xy32),imag(xy33)];

    case 7
        X=[real(ab22),real(ab32),real(ab33),real(ab13);
           imag(ab22),imag(ab32),imag(ab33),imag(ab13);
           real(xy22),real(xy32),real(xy33),real(xy13);
           imag(xy22),imag(xy32),imag(xy33),imag(xy13)];

    case 8
        X=[real(ab32),real(ab33),real(ab13),real(ab11);
           imag(ab32),imag(ab33),imag(ab13),imag(ab11);
           real(xy32),real(xy33),real(xy13),real(xy11);
           imag(xy32),imag(xy33),imag(xy13),imag(xy11)];

    case 9
        X=[real(ab33),real(ab13),real(ab11),real(ab51);
           imag(ab33),imag(ab13),imag(ab11),imag(ab51);
           real(xy33),real(xy13),real(xy11),real(xy51);
           imag(xy33),imag(xy13),imag(xy11),imag(xy51)];

    case 10
        X=[real(ab13),real(ab11),real(ab51),real(ab55);
           imag(ab13),imag(ab11),imag(ab51),imag(ab55);
           real(xy13),real(xy11),real(xy51),real(xy55);
           imag(xy13),imag(xy11),imag(xy51),imag(xy55)];

    case 11
        X=[real(ab11),real(ab51),real(ab55),real(ab45);
           imag(ab11),imag(ab51),imag(ab55),imag(ab45);
           real(xy11),real(xy51),real(xy55),real(xy45);
           imag(xy11),imag(xy51),imag(xy55),imag(xy45)];

    case 12
        X=[real(ab51),real(ab55),real(ab45),real(ab44);
           imag(ab51),imag(ab55),imag(ab45),imag(ab44);
           real(xy51),real(xy55),real(xy45),real(xy44);
           imag(xy51),imag(xy55),imag(xy45),imag(xy44)];

    otherwise
        X=[0,0,0,0;
           0,0,0,0;
           0,0,0,0;
           0,0,0,0];

end
Y=[Ualpha;Ubeta;Ux;Uy]*Tpwm;
T = X \ Y;

% t1=T(1);
% if t1<15e-6
%     t1=15e-6;
% end
% t2=T(2);
% if t2<15e-6
%     t2=15e-6;
% end
% t3=T(3);
% if t3<1e-6
%     t3=1e-6;
% end
% t4=T(4);
% if t4<1e-6
%     t4=1e-6;
% end

t1=T(1);
t2=T(2);
t3=T(3);
t4=T(4);
t1cp = 0;
t2cp = 0;
t3cp = 0;
t4cp = 0;
% if T(1) >= 0
%     t1 = T(1);
% else
%     t1 = 0;
%     t1cp = -T(1);
% end
% if T(2) >= 0
%     t2 = T(2);
% else
%     t2 = 0;
%     t2cp = -T(2);
% end
% if T(3) >= 0
%     t3 = T(3);
% else
%     t3 = 0;
%     t3cp = -T(3);
% end
% if T(4) >= 0
%     t4 = T(4);
% else
%     t4 = 0;
%     t4cp = -T(4);
% end

Tsum=t1+t2+t3+t4;
if Tsum>Tpwm
    t1=t1*Tpwm/Tsum;
    t2=t2*Tpwm/Tsum;
    t3=t3*Tpwm/Tsum;
    t4=t4*Tpwm/Tsum;
end
t0=Tpwm-t1-t2-t3-t4;
end

== matlab function DualSixPhaseInverter/SVPWM2/rest of others ==
  data: N input; T1 input; T2 input; T3 input; T4 input; T0 input; a1 output; a2 output; b1 output; b2 output; c1 output; c2 output; d1 output; d2 output; e1 output; e2 output; f1 output; f2 output; t1cp input; t2cp input; t3cp input; t4cp input
function [a1,a2,b1,b2,c1,c2,d1,d2,e1,e2,f1,f2] = fcn(N,T1,T2,T3,T4,T0,t1cp,t2cp,t3cp,t4cp)

%#xsxx
Ta=T0/4;
Tb=Ta+T2;
Tc=Tb+T1;
Td=Tc+T0/2;
Te=Td+T4;
Tf=Te+T3;

Ta1=T0/4;
Tb1=Ta1+T1;
Tc1=Tb1+T2;
Td1=Tc1+T0/2;
Te1=Td1+T3;
Tf1=Te1+T4;

%a1:phase A CMPA
%a2:phase A CMPB

a1 = 0;
a2 = 0;
b1 = 0;
b2 = 0;
c1 = 0;
c2 = 0;
d1 = 0;
d2 = 0;
e1 = 0;
e2 = 0;
f1 = 0;
f2 = 0;

if N==7
    a1=Ta;%TIme of "00" voltage vector 
    a2=Tf;%TIme of "48" voltage vector 
    d1=Ta;
    d2=Tf;
    b1=Tc;%TIme of "51" voltage vector 
    b2=Te + t1cp + t2cp + t3cp;%TIme of "56" voltage vector 
    e1=Tc;
    e2=Td + t1cp +t2cp +t3cp + t4cp;
    c1=Tb;%TIme of "49" voltage vector 
    c2=Td + t2cp + t3cp + t4cp;%TIme of "63" voltage vector 
    f1=Ta;
    f2=Td + t3cp + t4cp;
elseif N==8
    a1=Ta;
    a2=Tf;
    d1=Ta;
    d2=Tf;
    b1=Tc;
    b2=Tf + t1cp + t2cp;
    e1=Tc;
    e2=Te + t1cp + t2cp + t3cp;
    c1=Tc;
    c2=Td + t1cp + t2cp + t3cp + t4cp;
    f1=Tb;
    f2=Td + t2cp + t3cp + t4cp;
elseif N==9
    a1=Ta1;
    a2=Te1 + t4cp;
    d1=Ta1;
    d2=Tf1;
    b1=Tb1;
    b2=Tf1 + t1cp;
    e1=Tc1;
    e2=Tf1 + t1cp + t2cp;
    c1=Tc1;
    c2=Td1 + t1cp + t2cp + t3cp + t4cp;
    f1=Tc1;
    f2=Td1 + t1cp + t2cp + t3cp + t4cp;
elseif N==10
    a1=Ta1;
    a2=Td1 + t3cp + t4cp;
    d1=Ta1;
    d2=Te1 + t4cp;
    b1=Ta1;
    b2=Tf1;
    e1=Tb1;
    e2=Tf1 + t1cp;
    c1=Tc1;
    c2=Td1 + t1cp + t2cp + t3cp + t4cp;
    f1=Tc1;
    f2=Td1 + t1cp + t2cp + t3cp + t4cp;
elseif N==11
    a1=Tb;
    a2=Td + t2cp + t3cp + t4cp;
    d1=Ta;
    d2=Td + t3cp + t4cp;
    b1=Ta;
    b2=Tf;
    e1=Ta;
    e2=Tf;
    c1=Tc;
    c2=Te + t1cp + t2cp + t3cp;
    f1=Tc;
    f2=Td + t1cp + t2cp + t3cp + t4cp;
elseif N==12
    a1=Tc;
    a2=Td + t1cp + t2cp + t3cp + t4cp;
    d1=Tb;
    d2=Td + t2cp + t3cp + t4cp;
    b1=Ta;
    b2=Tf;
    e1=Ta;
    e2=Tf;
    c1=Tc;
    c2=Tf + t1cp + t2cp;
    f1=Tc;
    f2=Te + t1cp + t2cp + t3cp;
elseif N==1
    a1=Tc1;
    a2=Td1 + t1cp + t2cp + t3cp + t4cp;
    d1=Tc1;
    d2=Td1 + t1cp + t2cp + t3cp + t4cp;
    b1=Ta1;
    b2=Te1 + t4cp;
    e1=Ta1;
    e2=Tf1;
    c1=Tb1;
    c2=Tf1 + t1cp;
    f1=Tc1;
    f2=Tf1 + t1cp + t2cp;
elseif N==2
    a1=Tc1;
    a2=Td1 + t1cp + t2cp + t3cp + t4cp;
    d1=Tc1;
    d2=Td1 + t1cp + t2cp + t3cp + t4cp;
    b1=Ta1;
    b2=Td1 + t3cp + t4cp;
    e1=Ta1;
    e2=Te1 + t4cp;
    c1=Ta1;
    c2=Tf1;
    f1=Tb1;
    f2=Tf1 + t1cp;
elseif N==3
    a1=Tc;
    a2=Te + t1cp + t2cp + t3cp;
    d1=Tc;
    d2=Td + t1cp + t2cp + t3cp + t4cp;
    b1=Tb;
    b2=Td + t2cp + t3cp + t4cp;
    e1=Ta;
    e2=Td + t3cp + t4cp;
    c1=Ta;
    c2=Tf;
    f1=Ta;
    f2=Tf;
elseif N==4
    a1=Tc;
    a2=Tf + t1cp + t2cp;
    d1=Tc;
    d2=Te + t1cp + t2cp + t3cp;
    b1=Tc;
    b2=Td + t1cp + t2cp + t3cp + t4cp;
    e1=Tb;
    e2=Td + t2cp + t3cp + t4cp;
    c1=Ta;
    c2=Tf;
    f1=Ta;
    f2=Tf;
elseif N==5
    a1=Tb1;
    a2=Tf1 + t1cp;
    d1=Tc1;
    d2=Tf1 + t1cp + t2cp;
    b1=Tc1;
    b2=Td1 + t1cp + t2cp + t3cp + t4cp;
    e1=Tc1;
    e2=Td1 + t1cp + t2cp + t3cp + t4cp;
    c1=Ta1;
    c2=Te1 + t4cp;
    f1=Ta1;
    f2=Tf1;
elseif N==6
    a1=Ta1;
    a2=Tf1;
    d1=Tb1;
    d2=Tf1 + t1cp;
    b1=Tc1;
    b2=Td1 + t1cp + t2cp + t3cp + t4cp;
    e1=Tc1;
    e2=Td1 + t1cp + t2cp + t3cp + t4cp;
    c1=Ta1;
    c2=Td1 + t3cp + t4cp;
    f1=Ta1;
    f2=Te1 + t4cp;
end

== matlab function DualSixPhaseInverter/SVPWM1/rest of others ==
  data: N input; T1 input; T2 input; T3 input; T4 input; T0 input; a1 output; a2 output; b1 output; b2 output; c1 output; c2 output; d1 output; d2 output; e1 output; e2 output; f1 output; f2 output; t1cp input; t2cp input; t3cp input; t4cp input
function [a1,a2,b1,b2,c1,c2,d1,d2,e1,e2,f1,f2] = fcn(N,T1,T2,T3,T4,T0,t1cp,t2cp,t3cp,t4cp)

%#xsxx
Ta=T0/4;
Tb=Ta+T2;
Tc=Tb+T1;
Td=Tc+T0/2;
Te=Td+T4;
Tf=Te+T3;

Ta1=T0/4;
Tb1=Ta1+T1;
Tc1=Tb1+T2;
Td1=Tc1+T0/2;
Te1=Td1+T3;
Tf1=Te1+T4;

%a1:phase A CMPA
%a2:phase A CMPB

a1 = 0;
a2 = 0;
b1 = 0;
b2 = 0;
c1 = 0;
c2 = 0;
d1 = 0;
d2 = 0;
e1 = 0;
e2 = 0;
f1 = 0;
f2 = 0;

if N==1
    a1=Ta;%TIme of "00" voltage vector 
    a2=Tf;%TIme of "48" voltage vector 
    d1=Ta;
    d2=Tf;
    b1=Tc;%TIme of "51" voltage vector 
    b2=Te + t1cp + t2cp + t3cp;%TIme of "56" voltage vector 
    e1=Tc;
    e2=Td + t1cp +t2cp +t3cp + t4cp;
    c1=Tb;%TIme of "49" voltage vector 
    c2=Td + t2cp + t3cp + t4cp;%TIme of "63" voltage vector 
    f1=Ta;
    f2=Td + t3cp + t4cp;
elseif N==2
    a1=Ta;
    a2=Tf;
    d1=Ta;
    d2=Tf;
    b1=Tc;
    b2=Tf + t1cp + t2cp;
    e1=Tc;
    e2=Te + t1cp + t2cp + t3cp;
    c1=Tc;
    c2=Td + t1cp + t2cp + t3cp + t4cp;
    f1=Tb;
    f2=Td + t2cp + t3cp + t4cp;
elseif N==3
    a1=Ta1;
    a2=Te1 + t4cp;
    d1=Ta1;
    d2=Tf1;
    b1=Tb1;
    b2=Tf1 + t1cp;
    e1=Tc1;
    e2=Tf1 + t1cp + t2cp;
    c1=Tc1;
    c2=Td1 + t1cp + t2cp + t3cp + t4cp;
    f1=Tc1;
    f2=Td1 + t1cp + t2cp + t3cp + t4cp;
elseif N==4
    a1=Ta1;
    a2=Td1 + t3cp + t4cp;
    d1=Ta1;
    d2=Te1 + t4cp;
    b1=Ta1;
    b2=Tf1;
    e1=Tb1;
    e2=Tf1 + t1cp;
    c1=Tc1;
    c2=Td1 + t1cp + t2cp + t3cp + t4cp;
    f1=Tc1;
    f2=Td1 + t1cp + t2cp + t3cp + t4cp;
elseif N==5
    a1=Tb;
    a2=Td + t2cp + t3cp + t4cp;
    d1=Ta;
    d2=Td + t3cp + t4cp;
    b1=Ta;
    b2=Tf;
    e1=Ta;
    e2=Tf;
    c1=Tc;
    c2=Te + t1cp + t2cp + t3cp;
    f1=Tc;
    f2=Td + t1cp + t2cp + t3cp + t4cp;
elseif N==6
    a1=Tc;
    a2=Td + t1cp + t2cp + t3cp + t4cp;
    d1=Tb;
    d2=Td + t2cp + t3cp + t4cp;
    b1=Ta;
    b2=Tf;
    e1=Ta;
    e2=Tf;
    c1=Tc;
    c2=Tf + t1cp + t2cp;
    f1=Tc;
    f2=Te + t1cp + t2cp + t3cp;
elseif N==7
    a1=Tc1;
    a2=Td1 + t1cp + t2cp + t3cp + t4cp;
    d1=Tc1;
    d2=Td1 + t1cp + t2cp + t3cp + t4cp;
    b1=Ta1;
    b2=Te1 + t4cp;
    e1=Ta1;
    e2=Tf1;
    c1=Tb1;
    c2=Tf1 + t1cp;
    f1=Tc1;
    f2=Tf1 + t1cp + t2cp;
elseif N==8
    a1=Tc1;
    a2=Td1 + t1cp + t2cp + t3cp + t4cp;
    d1=Tc1;
    d2=Td1 + t1cp + t2cp + t3cp + t4cp;
    b1=Ta1;
    b2=Td1 + t3cp + t4cp;
    e1=Ta1;
    e2=Te1 + t4cp;
    c1=Ta1;
    c2=Tf1;
    f1=Tb1;
    f2=Tf1 + t1cp;
elseif N==9
    a1=Tc;
    a2=Te + t1cp + t2cp + t3cp;
    d1=Tc;
    d2=Td + t1cp + t2cp + t3cp + t4cp;
    b1=Tb;
    b2=Td + t2cp + t3cp + t4cp;
    e1=Ta;
    e2=Td + t3cp + t4cp;
    c1=Ta;
    c2=Tf;
    f1=Ta;
    f2=Tf;
elseif N==10
    a1=Tc;
    a2=Tf + t1cp + t2cp;
    d1=Tc;
    d2=Te + t1cp + t2cp + t3cp;
    b1=Tc;
    b2=Td + t1cp + t2cp + t3cp + t4cp;
    e1=Tb;
    e2=Td + t2cp + t3cp + t4cp;
    c1=Ta;
    c2=Tf;
    f1=Ta;
    f2=Tf;
elseif N==11
    a1=Tb1;
    a2=Tf1 + t1cp;
    d1=Tc1;
    d2=Tf1 + t1cp + t2cp;
    b1=Tc1;
    b2=Td1 + t1cp + t2cp + t3cp + t4cp;
    e1=Tc1;
    e2=Td1 + t1cp + t2cp + t3cp + t4cp;
    c1=Ta1;
    c2=Te1 + t4cp;
    f1=Ta1;
    f2=Tf1;
elseif N==12
    a1=Ta1;
    a2=Tf1;
    d1=Tb1;
    d2=Tf1 + t1cp;
    b1=Tc1;
    b2=Td1 + t1cp + t2cp + t3cp + t4cp;
    e1=Tc1;
    e2=Td1 + t1cp + t2cp + t3cp + t4cp;
    c1=Ta1;
    c2=Td1 + t3cp + t4cp;
    f1=Ta1;
    f2=Te1 + t4cp;
end
